simulink model "observerModel"  (Simulink 8.9)
settings: Solver=ode45  StartTime=0.0  StopTime=duration  RelTol=1e-5  AbsTol=1e-5  EnableMultiTasking=on
values from neighbouring files (symbols this model uses):
  delta_t = time(2) - time (1)    [observer_for_SOE1a.m]
  f_oto = handles.f_oto    [observer_for_SOE1a.m]
  f_scc = handles.f_scc    [observer_for_SOE1a.m]
  oto_a = 60*[1 1 1]'    [observer_for_SOE1a.m]
  oto_Ka = 1.3*[1 1 1]'    [observer_for_SOE1a.m]
  Q0 = [cos(E_angle/2) E(1)*sin(E_angle/2) E(2)*sin(E_angle/2) E(3)*sin(E_angle/2)]'    [observer_for_SOE1a.m]
  tau_a = handles.tau_a_value*[1 1 1]'    [observer_for_SOE1a.m]
  tau_scc = handles.tau_scc_value*[1 1 1]'    [observer_for_SOE1a.m]
undefined symbols (not defined in the file or in its folder): f_visO, f_visV, f_visX, kaa, kaaxy, kfg, kfw, kgvg, kwg, kwvw, kww, kxdotva, kxvv, x_leak, y_leak, z_leak
libraries: sharedutil x2
(part 3 of 3)

== system observerModel/Quaternion Rotator/Head to Limbic Angular Velocity Transform/Quaternion Integrator1/delta_q/Z ==
  q : Inport
  Constant : Constant
  Demux : Demux
  Product{,1..3} (4 alike) : Product  RndMeth=Zero
  Sum : Sum  Inputs=++++
  Sum1 : Sum  Inputs=+-
  z : Outport
  wires:
  Demux/1 -> Product/1, Product/2
  Demux/2 -> Product1/1, Product1/2
  Demux/3 -> Product2/1, Product2/2
  Demux/4 -> Product3/1, Product3/2
  q/1 -> Demux/1
  Product/1 -> Sum/1
  Product1/1 -> Sum/2
  Product2/1 -> Sum/3
  Product3/1 -> Sum/4
  Sum/1 -> Sum1/2
  Constant/1 -> Sum1/1
  Sum1/1 -> z/1

== system observerModel/Quaternion Rotator/Quaternion Integrator/delta_q/C/C1 ==
  omega : Inport
  q : Inport  Port=2
  Demux : Demux  Outputs=3
  Demux1 : Demux
  Gain : Gain  Gain=-0.5
  Product : Product  RndMeth=Zero
  Product1 : Product  RndMeth=Zero
  Product2 : Product  RndMeth=Zero
  Sum : Sum  Inputs=+++
  Terminator : Terminator
  c1 : Outport
  wires:
  Demux1/2 -> Product/2
  Demux/1 -> Product/1
  Demux1/3 -> Product1/2
  Demux/2 -> Product1/1
  Demux1/4 -> Product2/2
  Demux/3 -> Product2/1
  Product/1 -> Sum/1
  Product1/1 -> Sum/2
  Product2/1 -> Sum/3
  Sum/1 -> Gain/1
  omega/1 -> Demux/1
  Gain/1 -> c1/1
  q/1 -> Demux1/1
  Demux1/1 -> Terminator/1

== system observerModel/Quaternion Rotator/Quaternion Integrator/delta_q/C/C2 ==
  omega : Inport
  q : Inport  Port=2
  Demux : Demux  Outputs=3
  Demux1 : Demux
  Gain : Gain  Gain=0.5
  Product : Product  RndMeth=Zero
  Product1 : Product  RndMeth=Zero
  Product2 : Product  RndMeth=Zero
  Sum : Sum  Inputs=++-
  Terminator : Terminator
  c2 : Outport
  wires:
  Product/1 -> Sum/1
  Product1/1 -> Sum/2
  Product2/1 -> Sum/3
  Sum/1 -> Gain/1
  omega/1 -> Demux/1
  Gain/1 -> c2/1
  q/1 -> Demux1/1
  Demux1/1 -> Product/2
  Demux/1 -> Product/1
  Demux1/3 -> Product1/2
  Demux/3 -> Product1/1
  Demux1/4 -> Product2/2
  Demux/2 -> Product2/1
  Demux1/2 -> Terminator/1

== system observerModel/Quaternion Rotator/Quaternion Integrator/delta_q/C/C3 ==
  omega : Inport
  q : Inport  Port=2
  Demux : Demux  Outputs=3
  Demux1 : Demux
  Gain : Gain  Gain=0.5
  Product : Product  RndMeth=Zero
  Product1 : Product  RndMeth=Zero
  Product2 : Product  RndMeth=Zero
  Sum : Sum  Inputs=++-
  Terminator : Terminator
  c3 : Outport
  wires:
  Product/1 -> Sum/1
  Product1/1 -> Sum/2
  Product2/1 -> Sum/3
  Sum/1 -> Gain/1
  omega/1 -> Demux/1
  Gain/1 -> c3/1
  q/1 -> Demux1/1
  Demux1/1 -> Product/2
  Demux/2 -> Product/1
  Demux1/4 -> Product1/2
  Demux/1 -> Product1/1
  Demux1/2 -> Product2/2
  Demux/3 -> Product2/1
  Demux1/3 -> Terminator/1

== system observerModel/Quaternion Rotator/Quaternion Integrator/delta_q/C/C4 ==
  omega : Inport
  q : Inport  Port=2
  Demux : Demux  Outputs=3
  Demux1 : Demux
  Gain : Gain  Gain=0.5
  Product : Product  RndMeth=Zero
  Product1 : Product  RndMeth=Zero
  Product2 : Product  RndMeth=Zero
  Sum : Sum  Inputs=++-
  Terminator : Terminator
  c4 : Outport
  wires:
  Product/1 -> Sum/1
  Product1/1 -> Sum/2
  Product2/1 -> Sum/3
  Sum/1 -> Gain/1
  omega/1 -> Demux/1
  Gain/1 -> c4/1
  q/1 -> Demux1/1
  Demux1/1 -> Product/2
  Demux/3 -> Product/1
  Demux1/2 -> Product1/2
  Demux/2 -> Product1/1
  Demux1/3 -> Product2/2
  Demux/1 -> Product2/1
  Demux1/4 -> Terminator/1

== system observerModel/Quaternion Rotator2/Head to Limbic Angular Velocity Transform Rotation Matrix/Quaternion Integrator1/delta_q/C ==
  omega : Inport
  q : Inport  Port=2
  C1 : Subsystem
  C2 : Subsystem
  C3 : Subsystem
  C4 : Subsystem
  Mux : Mux
  C : Outport
  wires:
  omega/1 -> C1/1(omega), C2/1(omega), C3/1(omega), C4/1(omega)
  q/1 -> C4/2(q), C3/2(q), C2/2(q), C1/2(q)
  C1/1(c1) -> Mux/1
  C2/1(c2) -> Mux/2
  C3/1(c3) -> Mux/3
  C4/1(c4) -> Mux/4
  Mux/1 -> C/1

== system observerModel/Quaternion Rotator2/Head to Limbic Angular Velocity Transform Rotation Matrix/Quaternion Integrator1/delta_q/K ==
  Product : Product  RndMeth=Zero
  k : Constant  Value=1/delta_t
  value : Constant  Value=0.9
  K : Outport
  wires:
  k/1 -> Product/1
  Product/1 -> K/1
  value/1 -> Product/2

== system observerModel/Quaternion Rotator2/Head to Limbic Angular Velocity Transform Rotation Matrix/Quaternion Integrator1/delta_q/Z ==
  q : Inport
  Constant : Constant
  Demux : Demux
  Product{,1..3} (4 alike) : Product  RndMeth=Zero
  Sum : Sum  Inputs=++++
  Sum1 : Sum  Inputs=+-
  z : Outport
  wires:
  Demux/1 -> Product/1, Product/2
  Demux/2 -> Product1/1, Product1/2
  Demux/3 -> Product2/1, Product2/2
  Demux/4 -> Product3/1, Product3/2
  q/1 -> Demux/1
  Product/1 -> Sum/1
  Product1/1 -> Sum/2
  Product2/1 -> Sum/3
  Product3/1 -> Sum/4
  Sum/1 -> Sum1/2
  Constant/1 -> Sum1/1
  Sum1/1 -> z/1

== system observerModel/Quaternion Rotator2/Quaternion Integrator/delta_q/C/C1 ==
  omega : Inport
  q : Inport  Port=2
  Demux : Demux  Outputs=3
  Demux1 : Demux
  Gain : Gain  Gain=-0.5
  Product : Product  RndMeth=Zero
  Product1 : Product  RndMeth=Zero
  Product2 : Product  RndMeth=Zero
  Sum : Sum  Inputs=+++
  Terminator : Terminator
  c1 : Outport
  wires:
  Demux1/2 -> Product/2
  Demux/1 -> Product/1
  Demux1/3 -> Product1/2
  Demux/2 -> Product1/1
  Demux1/4 -> Product2/2
  Demux/3 -> Product2/1
  Product/1 -> Sum/1
  Product1/1 -> Sum/2
  Product2/1 -> Sum/3
  Sum/1 -> Gain/1
  omega/1 -> Demux/1
  Gain/1 -> c1/1
  q/1 -> Demux1/1
  Demux1/1 -> Terminator/1

== system observerModel/Quaternion Rotator2/Quaternion Integrator/delta_q/C/C2 ==
  omega : Inport
  q : Inport  Port=2
  Demux : Demux  Outputs=3
  Demux1 : Demux
  Gain : Gain  Gain=0.5
  Product : Product  RndMeth=Zero
  Product1 : Product  RndMeth=Zero
  Product2 : Product  RndMeth=Zero
  Sum : Sum  Inputs=++-
  Terminator : Terminator
  c2 : Outport
  wires:
  Product/1 -> Sum/1
  Product1/1 -> Sum/2
  Product2/1 -> Sum/3
  Sum/1 -> Gain/1
  omega/1 -> Demux/1
  Gain/1 -> c2/1
  q/1 -> Demux1/1
  Demux1/1 -> Product/2
  Demux/1 -> Product/1
  Demux1/3 -> Product1/2
  Demux/3 -> Product1/1
  Demux1/4 -> Product2/2
  Demux/2 -> Product2/1
  Demux1/2 -> Terminator/1

== system observerModel/Quaternion Rotator2/Quaternion Integrator/delta_q/C/C3 ==
  omega : Inport
  q : Inport  Port=2
  Demux : Demux  Outputs=3
  Demux1 : Demux
  Gain : Gain  Gain=0.5
  Product : Product  RndMeth=Zero
  Product1 : Product  RndMeth=Zero
  Product2 : Product  RndMeth=Zero
  Sum : Sum  Inputs=++-
  Terminator : Terminator
  c3 : Outport
  wires:
  Product/1 -> Sum/1
  Product1/1 -> Sum/2
  Product2/1 -> Sum/3
  Sum/1 -> Gain/1
  omega/1 -> Demux/1
  Gain/1 -> c3/1
  q/1 -> Demux1/1
  Demux1/1 -> Product/2
  Demux/2 -> Product/1
  Demux1/4 -> Product1/2
  Demux/1 -> Product1/1
  Demux1/2 -> Product2/2
  Demux/3 -> Product2/1
  Demux1/3 -> Terminator/1

== system observerModel/Quaternion Rotator2/Quaternion Integrator/delta_q/C/C4 ==
  omega : Inport
  q : Inport  Port=2
  Demux : Demux  Outputs=3
  Demux1 : Demux
  Gain : Gain  Gain=0.5
  Product : Product  RndMeth=Zero
  Product1 : Product  RndMeth=Zero
  Product2 : Product  RndMeth=Zero
  Sum : Sum  Inputs=++-
  Terminator : Terminator
  c4 : Outport
  wires:
  Product/1 -> Sum/1
  Product1/1 -> Sum/2
  Product2/1 -> Sum/3
  Sum/1 -> Gain/1
  omega/1 -> Demux/1
  Gain/1 -> c4/1
  q/1 -> Demux1/1
  Demux1/1 -> Product/2
  Demux/3 -> Product/1
  Demux1/2 -> Product1/2
  Demux/2 -> Product1/1
  Demux1/3 -> Product2/2
  Demux/1 -> Product2/1
  Demux1/4 -> Terminator/1

== system observerModel/Quaternion Rotator/Head to Limbic Angular Velocity Transform/Quaternion Integrator1/delta_q/C/C1 ==
  omega : Inport
  q : Inport  Port=2
  Demux : Demux  Outputs=3
  Demux1 : Demux
  Gain : Gain  Gain=-0.5
  Product : Product  RndMeth=Zero
  Product1 : Product  RndMeth=Zero
  Product2 : Product  RndMeth=Zero
  Sum : Sum  Inputs=+++
  Terminator : Terminator
  c1 : Outport
  wires:
  Demux1/2 -> Product/2
  Demux/1 -> Product/1
  Demux1/3 -> Product1/2
  Demux/2 -> Product1/1
  Demux1/4 -> Product2/2
  Demux/3 -> Product2/1
  Product/1 -> Sum/1
  Product1/1 -> Sum/2
  Product2/1 -> Sum/3
  Sum/1 -> Gain/1
  omega/1 -> Demux/1
  Gain/1 -> c1/1
  q/1 -> Demux1/1
  Demux1/1 -> Terminator/1

== system observerModel/Quaternion Rotator/Head to Limbic Angular Velocity Transform/Quaternion Integrator1/delta_q/C/C2 ==
  omega : Inport
  q : Inport  Port=2
  Demux : Demux  Outputs=3
  Demux1 : Demux
  Gain : Gain  Gain=0.5
  Product : Product  RndMeth=Zero
  Product1 : Product  RndMeth=Zero
  Product2 : Product  RndMeth=Zero
  Sum : Sum  Inputs=++-
  Terminator : Terminator
  c2 : Outport
  wires:
  Product/1 -> Sum/1
  Product1/1 -> Sum/2
  Product2/1 -> Sum/3
  Sum/1 -> Gain/1
  omega/1 -> Demux/1
  Gain/1 -> c2/1
  q/1 -> Demux1/1
  Demux1/1 -> Product/2
  Demux/1 -> Product/1
  Demux1/3 -> Product1/2
  Demux/3 -> Product1/1
  Demux1/4 -> Product2/2
  Demux/2 -> Product2/1
  Demux1/2 -> Terminator/1

== system observerModel/Quaternion Rotator/Head to Limbic Angular Velocity Transform/Quaternion Integrator1/delta_q/C/C3 ==
  omega : Inport
  q : Inport  Port=2
  Demux : Demux  Outputs=3
  Demux1 : Demux
  Gain : Gain  Gain=0.5
  Product : Product  RndMeth=Zero
  Product1 : Product  RndMeth=Zero
  Product2 : Product  RndMeth=Zero
  Sum : Sum  Inputs=++-
  Terminator : Terminator
  c3 : Outport
  wires:
  Product/1 -> Sum/1
  Product1/1 -> Sum/2
  Product2/1 -> Sum/3
  Sum/1 -> Gain/1
  omega/1 -> Demux/1
  Gain/1 -> c3/1
  q/1 -> Demux1/1
  Demux1/1 -> Product/2
  Demux/2 -> Product/1
  Demux1/4 -> Product1/2
  Demux/1 -> Product1/1
  Demux1/2 -> Product2/2
  Demux/3 -> Product2/1
  Demux1/3 -> Terminator/1

== system observerModel/Quaternion Rotator/Head to Limbic Angular Velocity Transform/Quaternion Integrator1/delta_q/C/C4 ==
  omega : Inport
  q : Inport  Port=2
  Demux : Demux  Outputs=3
  Demux1 : Demux
  Gain : Gain  Gain=0.5
  Product : Product  RndMeth=Zero
  Product1 : Product  RndMeth=Zero
  Product2 : Product  RndMeth=Zero
  Sum : Sum  Inputs=++-
  Terminator : Terminator
  c4 : Outport
  wires:
  Product/1 -> Sum/1
  Product1/1 -> Sum/2
  Product2/1 -> Sum/3
  Sum/1 -> Gain/1
  omega/1 -> Demux/1
  Gain/1 -> c4/1
  q/1 -> Demux1/1
  Demux1/1 -> Product/2
  Demux/3 -> Product/1
  Demux1/2 -> Product1/2
  Demux/2 -> Product1/1
  Demux1/3 -> Product2/2
  Demux/1 -> Product2/1
  Demux1/4 -> Terminator/1

== system observerModel/Quaternion Rotator2/Head to Limbic Angular Velocity Transform Rotation Matrix/Quaternion Integrator1/delta_q/C/C1 ==
  omega : Inport
  q : Inport  Port=2
  Demux : Demux  Outputs=3
  Demux1 : Demux
  Gain : Gain  Gain=-0.5
  Product : Product  RndMeth=Zero
  Product1 : Product  RndMeth=Zero
  Product2 : Product  RndMeth=Zero
  Sum : Sum  Inputs=+++
  Terminator : Terminator
  c1 : Outport
  wires:
  Demux1/2 -> Product/2
  Demux/1 -> Product/1
  Demux1/3 -> Product1/2
  Demux/2 -> Product1/1
  Demux1/4 -> Product2/2
  Demux/3 -> Product2/1
  Product/1 -> Sum/1
  Product1/1 -> Sum/2
  Product2/1 -> Sum/3
  Sum/1 -> Gain/1
  omega/1 -> Demux/1
  Gain/1 -> c1/1
  q/1 -> Demux1/1
  Demux1/1 -> Terminator/1

== system observerModel/Quaternion Rotator2/Head to Limbic Angular Velocity Transform Rotation Matrix/Quaternion Integrator1/delta_q/C/C2 ==
  omega : Inport
  q : Inport  Port=2
  Demux : Demux  Outputs=3
  Demux1 : Demux
  Gain : Gain  Gain=0.5
  Product : Product  RndMeth=Zero
  Product1 : Product  RndMeth=Zero
  Product2 : Product  RndMeth=Zero
  Sum : Sum  Inputs=++-
  Terminator : Terminator
  c2 : Outport
  wires:
  Product/1 -> Sum/1
  Product1/1 -> Sum/2
  Product2/1 -> Sum/3
  Sum/1 -> Gain/1
  omega/1 -> Demux/1
  Gain/1 -> c2/1
  q/1 -> Demux1/1
  Demux1/1 -> Product/2
  Demux/1 -> Product/1
  Demux1/3 -> Product1/2
  Demux/3 -> Product1/1
  Demux1/4 -> Product2/2
  Demux/2 -> Product2/1
  Demux1/2 -> Terminator/1

== system observerModel/Quaternion Rotator2/Head to Limbic Angular Velocity Transform Rotation Matrix/Quaternion Integrator1/delta_q/C/C3 ==
  omega : Inport
  q : Inport  Port=2
  Demux : Demux  Outputs=3
  Demux1 : Demux
  Gain : Gain  Gain=0.5
  Product : Product  RndMeth=Zero
  Product1 : Product  RndMeth=Zero
  Product2 : Product  RndMeth=Zero
  Sum : Sum  Inputs=++-
  Terminator : Terminator
  c3 : Outport
  wires:
  Product/1 -> Sum/1
  Product1/1 -> Sum/2
  Product2/1 -> Sum/3
  Sum/1 -> Gain/1
  omega/1 -> Demux/1
  Gain/1 -> c3/1
  q/1 -> Demux1/1
  Demux1/1 -> Product/2
  Demux/2 -> Product/1
  Demux1/4 -> Product1/2
  Demux/1 -> Product1/1
  Demux1/2 -> Product2/2
  Demux/3 -> Product2/1
  Demux1/3 -> Terminator/1

== system observerModel/Quaternion Rotator2/Head to Limbic Angular Velocity Transform Rotation Matrix/Quaternion Integrator1/delta_q/C/C4 ==
  omega : Inport
  q : Inport  Port=2
  Demux : Demux  Outputs=3
  Demux1 : Demux
  Gain : Gain  Gain=0.5
  Product : Product  RndMeth=Zero
  Product1 : Product  RndMeth=Zero
  Product2 : Product  RndMeth=Zero
  Sum : Sum  Inputs=++-
  Terminator : Terminator
  c4 : Outport
  wires:
  Product/1 -> Sum/1
  Product1/1 -> Sum/2
  Product2/1 -> Sum/3
  Sum/1 -> Gain/1
  omega/1 -> Demux/1
  Gain/1 -> c4/1
  q/1 -> Demux1/1
  Demux1/1 -> Product/2
  Demux/3 -> Product/1
  Demux1/2 -> Product1/2
  Demux/2 -> Product1/1
  Demux1/3 -> Product2/2
  Demux/1 -> Product2/1
  Demux1/4 -> Terminator/1
